simulink model "projet_ABS"  (R2017b)
settings: Solver=VariableStepAuto  StartTime=0.0  StopTime=10  RelTol=1e-3
InitFcn:
  | ABS_config
values from neighbouring files (symbols this model uses):
  f0 = 0.8    [ABS_config.m]
  m = 1000    [ABS_config.m]
  N = m*g/4    (= 2452.5)    [ABS_config.m]
  v0 = 100    [ABS_config.m]
libraries: simulink x1
settings Model: Creator=GEII Robot  LastModifiedBy=GEII Robot

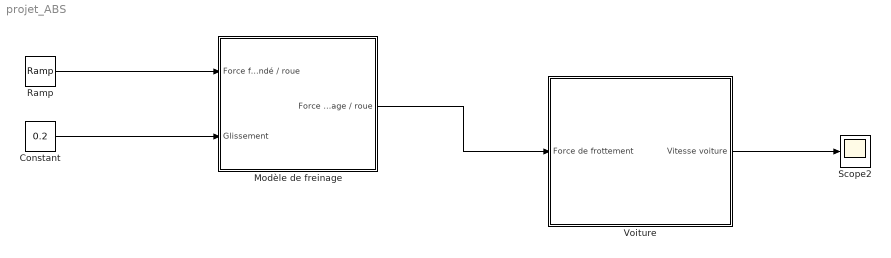
== system projet_ABS ==
  Constant : Constant  Value=0.2
  Modèle de freinage : Subsystem
  Ramp : simulink/Sources/Ramp  slope=f0*N/2  start=0  X0=0
  Scope2 : Scope
  Voiture : Subsystem
  wires:
  Constant/1 -> Modèle de freinage/2(Glissement)
  Ramp/1 -> Modèle de freinage/1(Force freinage demandé / roue)
  Modèle de freinage/1(Force de freinage / roue) -> Voiture/1(Force de frottement)
  Voiture/1(Vitesse voiture) -> Scope2/1

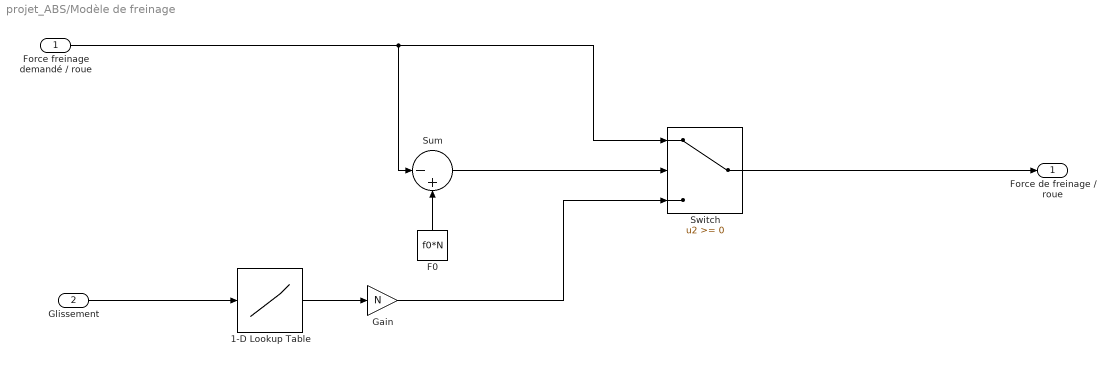
== system projet_ABS/Modèle de freinage ==
  Force freinage demandé / roue : Inport
  Glissement : Inport  Port=2
  1-D Lookup Table : Lookup_n-D  NumberOfTableDimensions=1  BreakpointsForDimension1=[0,0.025,0.05,0.1,0.15,0.2,0.25,0.3,0.35,0.4,0.45,0.5,0.55,0.6,0.65,0.7,0.75,0.8,0.85,0.9,0.95,1]  Table=[0,0.34,0.6,0.86,0.91,0.86,0.83,0.76,0.72,0.71,0.7,0.68,0.67,0.66,0.65,0.64,0.63,0.63,0.62,0.615,0.61,0.61]  InternalRulePriority=Speed  RndMeth=Simplest  InputSameDT=on
  F0 : Constant  Value=f0*N
  Gain : Gain  Gain=N
  Sum : Sum  Inputs=|-+
  Switch : Switch
  Force de freinage / roue : Outport
  wires:
  Glissement/1 -> 1-D Lookup Table/1
  Force freinage demandé / roue/1 -> Sum/1, Switch/1
  1-D Lookup Table/1 -> Gain/1
  Switch/1 -> Force de freinage / roue/1
  Gain/1 -> Switch/3
  Sum/1 -> Switch/2
  F0/1 -> Sum/2

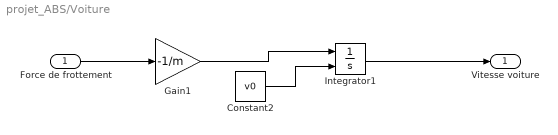
== system projet_ABS/Voiture ==
  Force de frottement : Inport
  Constant2 : Constant  Value=v0
  Gain1 : Gain  Gain=-1/m
  Integrator1 : Integrator  InitialConditionSource=external
  Vitesse voiture : Outport
  wires:
  Gain1/1 -> Integrator1/1
  Constant2/1 -> Integrator1/2
  Integrator1/1 -> Vitesse voiture/1
  Force de frottement/1 -> Gain1/1
